simulink subsystem "ControladorBA"  (R2023b)
settings: Solver=VariableStepAuto  StartTime=0.0  StopTime=10.0  RelTol=1e-3
settings Model: Creator=jaime  LastModifiedBy=jaime

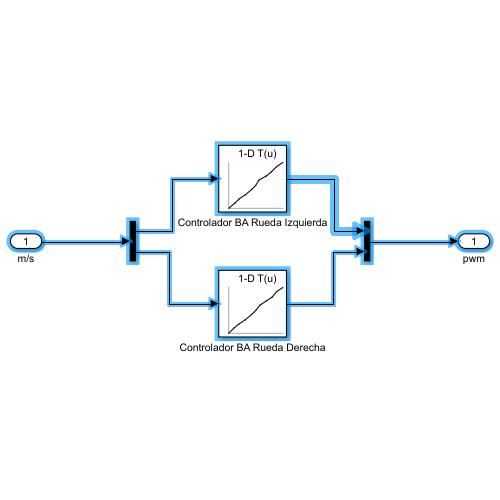
[thumbnail: Simulink's stored preview of the top-level diagram]
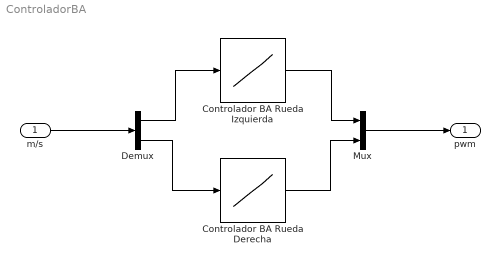
== system ControladorBA ==
  m/s : Inport
  Controlador BA Rueda Derecha : Lookup_n-D  NumberOfTableDimensions=1  BreakpointsForDimension1=[-0.477911025285721 -0.37655571103096 -0.289655953645706 -0.188268885016441 -0.07241202890873 0 0.072412684559822 0.188272625207901 0.28964364528656 0.376543760299683 0.477922409772873]  Table=[-255 -200 -150 -100 -50 0 50 100 150 200 255]  InternalRulePriority=Speed  RndMeth=Simplest
  Controlador BA Rueda Izquierda : Lookup_n-D  NumberOfTableDimensions=1  BreakpointsForDimension1=[-0.463433384895325 -0.362071424722672 -0.275177627801895 -0.173785284161568 -0.072406068444252 0 0.057930134236813 0.173790171742439 0.275161534547806 0.362062811851501 0.463441461324692]  Table=[-255 -200 -150 -100 -50 0 50 100 150 200 255]  InternalRulePriority=Speed  RndMeth=Simplest
  Demux : Demux  Outputs=2
  Mux : Mux  Inputs=2
  pwm : Outport
  wires:
  Controlador BA Rueda Derecha/1 -> Mux/2
  Demux/1 -> Controlador BA Rueda Izquierda/1
  Demux/2 -> Controlador BA Rueda Derecha/1
  Mux/1 -> pwm/1
  m/s/1 -> Demux/1
  Controlador BA Rueda Izquierda/1 -> Mux/1
